simulink model "RealModel"  (R2018a)
settings: Solver=VariableStepAuto  StartTime=0.0  StopTime=10.0  RelTol=1e-3
settings Model: Creator=Administrator  LastModifiedBy=Administrator

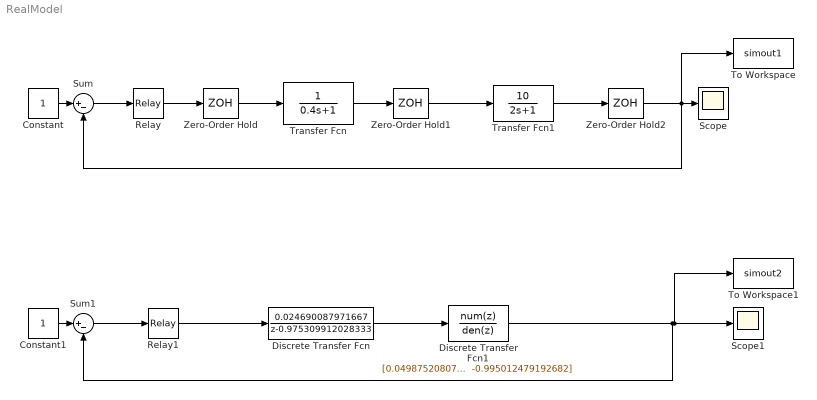
== system RealModel ==
  Constant : Constant
  Constant1 : Constant
  Discrete Transfer Fcn : DiscreteTransferFcn  Numerator=[0.024690087971667]  Denominator="[1.000000000000000  -0.975309912028333]"  SampleTime=0.01
  Discrete Transfer Fcn1 : DiscreteTransferFcn  Numerator=[0.049875208073177]  Denominator="[1.000000000000000  -0.995012479192682]"  SampleTime=0.01
  Relay : Relay  OnSwitchValue=0.1  OffSwitchValue=-0.1  OffOutputValue=-1
  Relay1 : Relay  OnSwitchValue=0.1  OffSwitchValue=-0.1  OffOutputValue=-1
  Scope : Scope
  Scope1 : Scope
  Sum : Sum  Inputs=|+-
  Sum1 : Sum  Inputs=|+-
  To Workspace : ToWorkspace  VariableName=simout1  SaveFormat=Timeseries  SampleTime=-1
  To Workspace1 : ToWorkspace  VariableName=simout2  SaveFormat=Timeseries  SampleTime=-1
  Transfer Fcn : TransferFcn  Denominator=[0.4 1]
  Transfer Fcn1 : TransferFcn  Numerator=[10]  Denominator=[2 1]
  Zero-Order Hold : ZeroOrderHold  SampleTime=0.01
  Zero-Order Hold1 : ZeroOrderHold  SampleTime=0.01
  Zero-Order Hold2 : ZeroOrderHold  SampleTime=0.01
  wires:
  Constant/1 -> Sum/1
  Zero-Order Hold/1 -> Transfer Fcn/1
  Transfer Fcn/1 -> Zero-Order Hold1/1
  Transfer Fcn1/1 -> Zero-Order Hold2/1
  Zero-Order Hold2/1 -> Sum/2, To Workspace/1, Scope/1
  Zero-Order Hold1/1 -> Transfer Fcn1/1
  Relay1/1 -> Discrete Transfer Fcn/1
  Sum1/1 -> Relay1/1
  Constant1/1 -> Sum1/1
  Discrete Transfer Fcn/1 -> Discrete Transfer Fcn1/1
  Discrete Transfer Fcn1/1 -> Sum1/2, To Workspace1/1, Scope1/1
  Sum/1 -> Relay/1
  Relay/1 -> Zero-Order Hold/1
